simulink model "sim_reg_position"  (R2025b)
settings: Solver=VariableStepAuto  StartTime=0.0  StopTime=10.0  RelTol=1e-3
undefined symbols (not defined in the file): setpoints, sim_trajectory_id
settings Model: Creator=Utente  LastModifiedBy=Utente

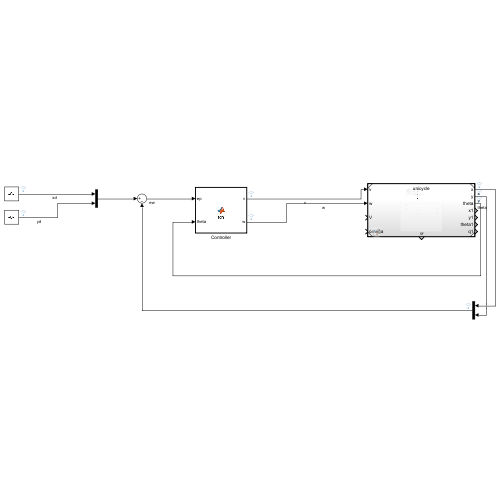
[thumbnail: Simulink's stored preview of the top-level diagram]
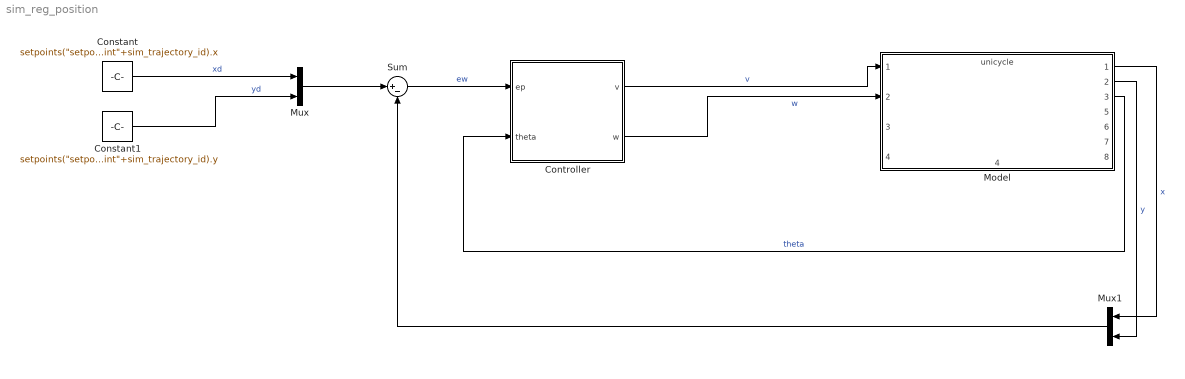
== system sim_reg_position ==
  Constant : Constant  Value="setpoints(\"setpoint\"+sim_trajectory_id).x"
  Constant1 : Constant  Value="setpoints(\"setpoint\"+sim_trajectory_id).y"
  Controller : MATLAB Function  TreatAsAtomicUnit=on
  Model : ModelReference  ModelNameDialog=unicycle.slx  SimulationMode=Normal  ModelReferenceVersion=1.12
      settings: PortSchema="{\"entries\":[{\"content\":{\"sides\":[{\"content\":{\"connectorIds\":[\"In1\",\"In2\",\"In3\",\"In4\"]},\"type\":\"ConnectorPlacement.EquallySpacedRectSide\",\"uuid\":\"ad25d81c-9301-4260-b0e7-6964e2a4144d\"},{\"content\":{\"connectorIds\":[\"Out1\",\"Out2\",\"Out3\",\"Out5\",\"Out6\",\"Out7\",\"Out8\"],\"side\":\"RIGHT\"},\"type\":\"ConnectorPlacement.EquallySpacedRectSide\",\"uuid\":\"e119e278-1a19-4d21-ac57-f30b4b2846c4\"},{\"content\":{\"side\":\"TOP\"},\"type\":\"ConnectorPlacement.EquallySpacedRectSide\",\"uuid\":\"f58ebd06-2844-4b35-9f44-2944c544d228\"},{\"content\":{\"connectorIds\":[\"Out4\"],\"side\":\"BOTTOM\"},\"type\":\"ConnectorPlacement.EquallySpacedRectSide\",\"uuid\":\"e9666c6b-2f60-424a-96df-bac3fd1a20e8\"}]},\"type\":\"ConnectorPlacement.EquallySpacedConnector\",\"uuid\":\"feeb8aec-4c5e-4f88-9f0a-836c4fc89b7c\"}],\"packageUris\":[\"http://schema.mathworks.com/mf0/Connector/R2020b\"],\"version\":\"1.0\"}"
  Mux : Mux  Inputs=2
  Mux1 : Mux  Inputs=2
  Sum : Sum  Inputs=|+-
  wires:
  Mux1/1 -> Sum/2
  Model/1 -> Mux1/1  "x"
  Model/2 -> Mux1/2  "y"
  Mux/1 -> Sum/1
  Sum/1 -> Controller/1(ep)  "ew"
  Model/3 -> Controller/2(theta)  "theta"
  Controller/1(v) -> Model/1  "v"
  Controller/2(w) -> Model/2  "w"
  Constant/1 -> Mux/1  "xd"
  Constant1/1 -> Mux/2  "yd"

== matlab function sim_reg_position/Controller ==
  data: ep input; v output; w output; theta input
function [v, w]= fcn(ep,theta)
x = -ep(1);
y = -ep(2);
theta = wrapToPi(theta);
epn = x*cos(theta) + y*sin(theta);
gamma = atan2(y, x) + pi - theta;
kv = 10;
kw = 20;
v = -kv * epn;
w = kw * gamma;
end
